simulink model "rotation_b"  (R2020a)
settings: Solver=VariableStepAuto  StartTime=0.0  StopTime=1000  RelTol=1e-3
values from neighbouring files (symbols this model uses):
  euler_angles_NfromB_0_deg = [0; 0; 0]    [p1partApartI.m]
  omega_BwrtN_rps = deg2rad([0; 0; 0.01])    [p1partApartI.m]
libraries: coordinate_transforms x1
settings Model: Creator=Nikita  LastModifiedBy=Nikita

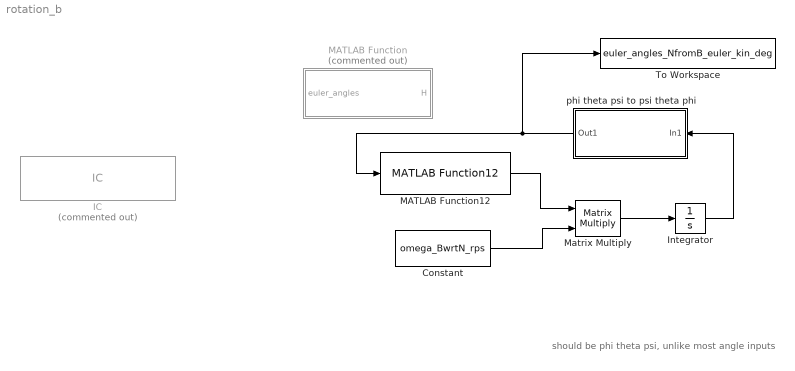
== system rotation_b ==
  note: should be phi theta psi, unlike most angle inputs
  Constant : Constant  Value=omega_BwrtN_rps
  IC : InitialCondition  Commented=on  Value=euler_angles_NfromB_0_deg
  Integrator : Integrator  InitialCondition=euler_angles_NfromB_0_deg
  MATLAB Function : MATLAB Function  Commented=on  TreatAsAtomicUnit=on
  MATLAB Function12 : coordinate_transforms/MATLAB Function12  SystemSampleTime=-1  Latency=0  AutoFrameSizeCalculation=off
  Matrix Multiply : Product  Multiplication=Matrix(*)
  To Workspace : ToWorkspace  VariableName=euler_angles_NfromB_euler_kin_deg  SampleTime=-1
  phi theta psi to psi theta phi : Subsystem
  wires:
  Constant/1 -> Matrix Multiply/2
  Matrix Multiply/1 -> Integrator/1
  Integrator/1 -> phi theta psi to psi theta phi/1(In1)
  MATLAB Function12/1 -> Matrix Multiply/1
  phi theta psi to psi theta phi/1(Out1) -> To Workspace/1, MATLAB Function12/1

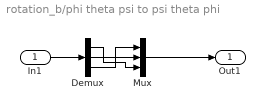
== system rotation_b/phi theta psi to psi theta phi ==
  In1 : Inport
  Demux : Demux  Outputs=3
  Mux : Mux  Inputs=3
  Out1 : Outport
  wires:
  Demux/3 -> Mux/1
  In1/1 -> Demux/1
  Demux/1 -> Mux/3
  Demux/2 -> Mux/2
  Mux/1 -> Out1/1

== matlab function rotation_b/MATLAB Function ==
  data: euler_angles input; H output
function H = angles2H(euler_angles)

psi     = euler_angles(1);
theta   = euler_angles(2);
phi     = euler_angles(3);

H = [1,    0,          -sin(theta);
     0, cos(phi),   sin(phi)*cos(theta);
     0, -sin(phi),  cos(phi)*cos(theta)];
